simulink subsystem "PvtSubSys_VSM_HWA"  (R2020b)
settings: Solver=VariableStepAuto  StartTime=0.0  StopTime=10.0  RelTol=1e-3
values from neighbouring files (symbols this model uses):
  P_VSM_HWA_ALCStsSW = 1    [HWA.sldd]
  P_VSM_HWA_DMS_Enable = 0.0    [HWA.sldd]
  P_VSM_HWA_EHR_Enable = 0.0    [HWA.sldd]
  P_VSM_HWAActivation_NOAMOd_Spd = 5.0    [HWA.sldd]
  P_VSM_HWAActivation_Spd_Low = 5.0    [HWA.sldd]
  P_VSM_HWAActivation_Spd_Up = 120.0    [HWA.sldd]
  P_VSM_NOH_PilotSelc_SW = 0.0    [HWA.sldd]
  P_VSM_NOH_Swt_Req_SW = 0.0    [HWA.sldd]
  P_VSM_TJA_PassSBRSpdExistSlow = 30.0    [HWA.sldd]
undefined symbols (not defined in the file or in its folder): ACC_STATE, P_VSM_PassSBRSpdIPLimt, TJA_STATE
libraries: simulink x65, TrueDurationTime x14
(part 2 of 2)

== stateflow chart PvtSubSys_VSM_HWA/Subsystem/HWA_SM/TJA ==
  state TJA_Main [parallel]
    settings: executionOrder=1
    state Off
      en:
      TJASts=TJA_Off;
    state TJAOn
      state Error
        en:
        TJASts=TJA_Error;
      state W
        state Ready
          en:
          TJASts=TJA_Ready;
        state Idle
          en:
          TJASts=TJA_Idle;
        state Active
          en:
          TJAActive=true;
          ex:
          TJAActive=false;
          state Active
            en:
            TJASts=TJA_Active;
            cnt=0;
            du:
            cnt=min(10,cnt+1)
          state SafeStop
            en:
            TJASts=TJA_SafeStop;
            du:
            SafeStopNum=min(300,SafeStopNum+1);
            TJASafeStopExit_b=(SafeStopNum>250);
            ACCParkShiftReq_b=VehicleStandstill;
            ex:
            TJAStopExit=true;
            ACCParkShiftReq_b=false;
            SafeStopNum=0;
          state Slow
            en:
            TJASts=TJA_SlowRetreat;
            ex:
            TJASlowExistReason = 0;
          TJA_Main.TJAOn.W.Active.Active -> SafeStop [order 1] : [TJASafeStopEn_b==true]
          Slow -> SafeStop [order 1] : [TJASafeStopEn_b==true]
          (junction 704) -> TJA_Main.TJAOn.W.Active.Active
          Slow -> (junction 704) [order 2] : [(PassSBROn ==1&&TJASlowExistReason == 2)||...
              | (Vego_kmh<=P_VSM_TJA_PassSBRSpdExistSlow&&TJASlowExistReason == 2)]
          TJA_Main.TJAOn.W.Active.Active -> (junction 701) [order 2] : [TJASlowExit_b==true]{TJASlowExistReason = 1;}
          (junction 701) -> Slow
          TJA_Main.TJAOn.W.Active.Active -> (junction 701) [order 3] : [TJAExit_PassSBR==1]{TJASlowExistReason = 2;}
        state Wait
          en:
          TJASts=TJA_Wait;
        (junction 438) -> Idle [order 1] : [(ACCSts==ACC_Reject)||...
            | (TJA_LCKState~=LCK_STATE.LCK_Active)||...
            | (TJASafeStopExit_b==true)||...
            | (ESSState==4||ESSState==5)||...
            | TJAError~=0]
        (junction 438) -> Ready [order 2] : [(ACCSts~=ACC_Reject)&&...
            | (TJA_LCKState==LCK_STATE.LCK_Active)&&...
            | (TJASafeStopExit_b==false)]
        Ready -> Idle [order 2] : [(ACCSts==ACC_Reject)||...
            | (TJA_LCKState~=LCK_STATE.LCK_Active)||...
            | TJAError~=0]
        Ready -> TJA_Main.TJAOn.W.Active.Active [order 1] : [Switch_SetTJA==true]
        Idle -> Ready : [(ACCSts~=ACC_Reject)&&...
            | (TJA_LCKState==LCK_STATE.LCK_Active)&&...
            | (TJASafeStopExit_b==false)&&...
            | (ESSState~=4&&ESSState~=5)&&...
            | TJAError==0]
        TJA_Main.TJAOn.W.Active.Active -> Wait [order 4] : [LCKSTS~=LCK_STATE.LCK_Active&&...
            | cnt>2]
        Wait -> Idle [order 1] : [ACCSts==ACC_STATE.ACC_Reject]
        Wait -> TJA_Main.TJAOn.W.Active.Active [order 2] : [LCKSTS==LCK_STATE.LCK_Active && TJASlowExit_b==false && TJAFastExit_b==false]
        (junction 697) -> Wait [order 1] : [TJASafeStopExit_b==false]
        TJA_Main.TJAOn.W.Active -> (junction 697) [order 1] : [TJAFastExit_b]
        (junction 697) -> Idle [order 2] : [TJASafeStopExit_b==true]
        TJA_Main.TJAOn.W.Active -> Idle [order 2] : [(ACCSts==ACC_Reject)||...
            | (ESSState==4||ESSState==5)]
      Error -> (junction 521) : [TJAError~=1]
      (junction 521) -> (junction 464)
      (junction 464) -> Error [order 1] : [TJAError==1]
      (junction 464) -> (junction 438) [order 2]
      W -> Error : [TJAError==1]
    (default) -> Off
    TJAOn -> Off : [(TJA_ON==false)||(VehConfigTJA==0)]
    Off -> (junction 521) : [(TJA_ON==true)&&(VehConfigTJA==1)]
  state P_SafeStopExit [parallel]
    settings: executionOrder=2
    state noP
    state P
      en:
      TJASafeStopExit_b=false;
    (default) -> noP
    noP -> P : [(TGS_LEVER==0)&&(TJASafeStopExit_b==true)]
    P -> noP : [TGS_LEVER~=0]
  data: TJA_ON input boolean size=1; ActiveNum local uint16 size=1 [0..100] =0; TJASts output Enum: TJA_STATE size=1 =TJA_STATE.TJA_Off; TJASafeStopExit_b output boolean size=1 =false; LCKSTS input Enum: LCK_STATE size=1; TJAStopExit local boolean size=1 =false; ACCParkShiftReq_b output boolean size=1 =0; HandsOff_b input boolean size=1 =false; VehConfigTJA input boolean; Switch_SetTJA input boolean; TGS_LEVER input; ActiveWaitNum local uint16 size=1; ESSState input; TJA_LCKState input; P_VSM_TJA_ActiveWaitNum parameter uint16; SafeStopNum local uint16; ACCSts input Enum: ACC_STATE; TJASlowExit_b input boolean; TJAFastExit_b input boolean; TJASafeStopEn_b input boolean; VehicleStandstill input boolean; cnt local uint16; Vego_kmh input uint8; TJAActive output boolean; TJAError input uint8; PassSBROn input; TJAExit_PassSBR input; TJASlowExistReason local uint8; P_VSM_TJA_PassSBRSpdExistSlow input

== stateflow chart PvtSubSys_VSM_HWA/Subsystem/HWA_SM/NOH ==
  state NOH
    state NOH_P
      state off
        en:
        NOHActiveNum=0;
        NOHSts = uint8(0);
      state P
        state Standby
          en:
          NOHSts = uint8(2);
        state Passive
          en:
          NOHSts = uint8(1);
        (default) -> Passive
        Passive -> Standby : [HWAActive == true&&PilotSts ~= 0]
        Standby -> Passive [order 1] : [HWAActive == false||PilotSts == 0]
      (default) -> off
      off -> P : [NOH_On==true]
      P -> off : [NOH_On==false]
    state Failure
    state NOH_Active
      en:
      NOHActiveNum = uint8(1);
      state Standstill
        en:
        NOHSts = uint8(6);
      state Slowretrate
        en:
        NOHSts = uint8(5);
      state Active
        en:
        NOHSts = uint8(3);
      state Override
        en:
        NOHSts = uint8(4);
      Standstill -> Override [order 2] : [ACCSts==ACC_Override]
      (junction 24) -> Standstill [order 2]
      Active -> Standstill [order 1] : [ACCSts==ACC_StandActive]
      Standstill -> Active [order 1] : [ACCSts==ACC_ActiveControl]
      (default) -> (junction 21)
      (junction 21) -> (junction 24) [order 2]
      (junction 21) -> Override [order 1] : [ACCSts==ACC_Override]
      Active -> Slowretrate [order 2] : [TJASts==TJA_SlowRetreat]
      (junction 24) -> Active [order 1] : [VehicleStandstill==0]
      Active -> Override [order 3] : [ACCSts==ACC_Override]
      Override -> Active : [ACCSts==ACC_ActiveControl]
    (default) -> NOH_P
    NOH_Active -> off [order 1] : [NOH_On==false]
    NOH_P -> Failure : [TJAError==1||HWAError==1]
    Failure -> NOH_P : [TJAError~=1&&HWAError~=1]
    NOH_Active -> Failure [order 2] : [TJAError==1||HWAError==1]
    Standby -> (junction 37) [order 2] : [NOH_Act==true]
    Standby -> (junction 37) [order 3] : [NOHActiveNum>0]
    NOH_Active -> P [order 3] : [HWAActive == false||PilotSts == 0]
    (junction 37) -> NOH_Active
  (default) -> NOH
  data: TJAError input uint8; HWAError input uint8; NOH_On input boolean; NOH_Act input boolean; PilotSts input uint8; ACCSts input Enum: ACC_STATE; TJASts input Enum: TJA_STATE; HWAActive input; VehicleStandstill input; NOHSts output; NOHActiveNum output uint8

== stateflow chart PvtSubSys_VSM_HWA/Subsystem/HWA_SM/HWA ==
  state Off
    en:
    HWASts=HWA_Off;
  state On
    state Passive
      state Ready [commented out]
        en:
        HWASts=HWA_Ready;
      state Idle
        en:
        HWASts=HWA_Idle;
      (default) -> Idle
      Ready -> Idle [commented out] : [TJASts~=TJA_STATE.TJA_Active]
      Idle -> Ready [commented out]
    state Active
      en:
      HWAActive=true;
      ex:
      HWAActive=false;
      state ActiveControl
        state a
          state LeftTurn
            en:
            HWASts=HWA_LeftTurn;
          state CC
            du:
            HWASts=HWA_CCAct;
          state RightTurn
            en:
            HWASts=HWA_RightTurn;
          CC -> LeftTurn [order 1] : [ALC_sts==2]
          LeftTurn -> (junction 662) : [ALC_sts==1]
          (junction 662) -> CC
          (default) -> CC
          RightTurn -> (junction 662) : [ALC_sts==1]
          CC -> RightTurn [order 2] : [ALC_sts==3]
        (default) -> a
    (default) -> Passive
    Passive -> ActiveControl : [TJASts==TJA_STATE.TJA_Active...
        | &&HWAerror==uint8(0)]
    ActiveControl -> Passive : [TJASts~=TJA_STATE.TJA_Active...
        | || HWAerror~=uint8(0)]
  (default) -> Off
  Off -> On : [TJA_ON==true]
  On -> Off : [TJA_ON==false]
  data: HWAerror input; TJA_ON input boolean; ALC_sts input uint8; ALC_LeTurnReq input uint8; ALC_RiTurnReq input uint8; HWA_LaneChangeEnable_Con input; HWA_LaneChangeDisable_Con input; HWASts output Enum: HWA_STATE =HWA_STATE.HWA_Off; HWAActive output boolean =false; ACCSts input =0; TJASts input Enum: TJA_STATE
